simulink model "pct23_mpc_ref_tracking_anti_windup_notworking"  (R2020b)
settings: Solver=FixedStepAuto  StartTime=0.0  StopTime=6000  FixedStep=Ts  RelTol=1e-3
values from neighbouring files (symbols this model uses):
  cit = cit{1}    [mpc_init.m]    (also in mpc_init_reference_tracking_tunable.m; ref_tracking1.mat = [0 0.565401791493]; ref_tracking10.mat = [0 0.565401791493]; ref_tracking11.mat = [0 0.565401791493])
  men = men{1}    [mpc_init.m]    (also in mpc_init_reference_tracking_tunable.m; ref_tracking1.mat = [1 -0.434598208507]; ref_tracking10.mat = [1 -0.434598208507]; ref_tracking11.mat = [1 -0.434598208507])
  Ts = 0.5    [mpc_init.m]    (also in mpc_init_reference_tracking_tunable.m; mpc_modif.m = 1; mpc_original.m; ref_tracking1.mat)
  ts = 0.5    [mpc_init.m]    (also in mpc_init_reference_tracking_tunable.m = 1; mpc_modif.m = 1; mpc_original.m = 1; ref_tracking1.mat)
  us = 35    [mpc_init.m]    (also in mpc_init_reference_tracking_tunable.m; mpc_modif.m = 50; mpc_original.m = 50; ref_tracking1.mat)
  ys = 35    [mpc_init.m]    (also in mpc_init_reference_tracking_tunable.m; mpc_modif.m; mpc_original.m; ref_tracking1.mat)
undefined symbols (not defined in the file or in its folder): MPC_fcn_yref
libraries: pid_lib x1, pct23_lib x1
settings Model: EnablePacing=on  Creator=belko  LastModifiedBy=lgalc

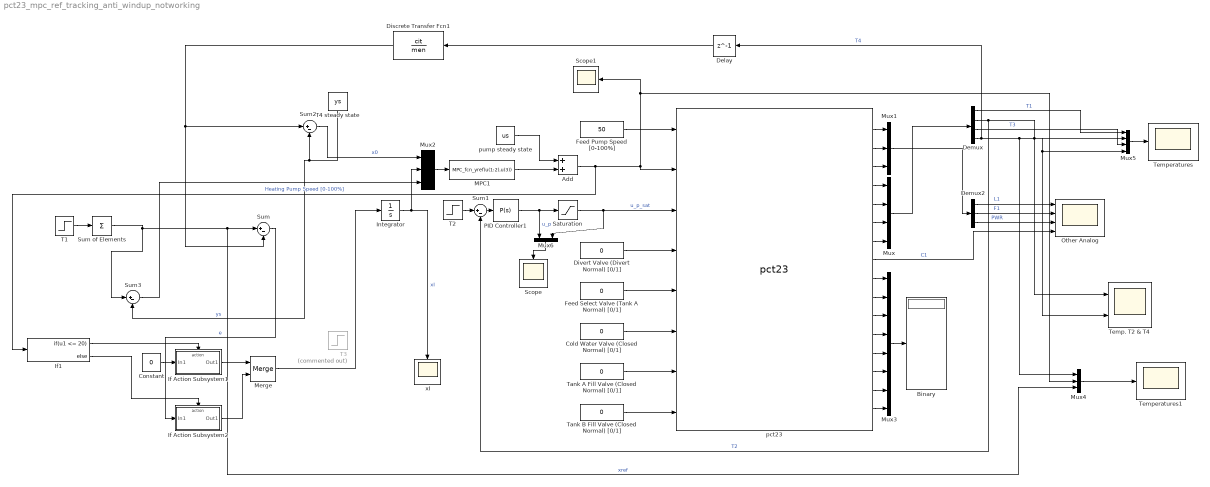
== system pct23_mpc_ref_tracking_anti_windup_notworking ==
  Add : Sum
  Binary : Display
  Cold Water Valve (Closed Normal) [0/1] : Constant  Value=0
  Constant : Constant  Value=0
  Delay : Delay  DelayLength=1  InitialCondition=ys  SampleTime=Ts
  Demux : Demux
  Demux2 : Demux  Outputs=3
  Discrete Transfer Fcn1 : DiscreteTransferFcn  Numerator=cit  Denominator=men  SampleTime=Ts
  Divert Valve (Divert Normal) [0/1] : Constant  Value=0
  Feed Pump Speed [0-100%] : Constant  Value=50
  Feed Select Valve (Tank A Normal) [0/1] : Constant  Value=0
  If Action Subsystem1 : Subsystem  TreatAsAtomicUnit=on
  If Action Subsystem2 : Subsystem  TreatAsAtomicUnit=on
  If1 : If  IfExpression=u1 <= 20
  Integrator : Integrator
  MPC1 : MATLABFcn  MATLABFcn=MPC_fcn_yref(u(1:2),u(3))  SampleTime=ts
  Merge : Merge  InitialOutput=0
  Mux : Mux
  Mux1 : Mux  Inputs=3
  Mux2 : Mux  Inputs=3
  Mux3 : Mux  Inputs=8
  Mux4 : Mux  Inputs=3
  Mux5 : Mux
  Mux6 : Mux  Inputs=2
  Other Analog : Scope  NumInputPorts=4
  PID Controller1 : pid_lib/PID Controller  Controller=P  Form=Parallel  TimeDomain=Continuous-time  UseExternalTs=off  SampleTime=-1  IntegratorMethod=Forward Euler  FilterMethod=Forward Euler  ControllerParametersSource=internal  P=20  I=1  D=0  UseFilter=on  N=100  TunerSelectOption=Transfer Function Based (PID Tuner App)  InitialConditionSource=internal  InitialConditionForIntegrator=0  InitialConditionForFilter=0  DifferentiatorICPrevScaledInput=0  ExternalReset=none  TrackingMode=off  Kt=1  LimitOutput=off  SatLimitsSource=internal  UpperSaturationLimit=inf  LowerSaturationLimit=-inf  LinearizeAsGain=on  AntiWindupMode=none  Kb=1  POutMin=[]  POutMax=[]  IOutMin=[]  IOutMax=[]  DOutMin=[]  DOutMax=[]  NOutMin=[]  NOutMax=[]  SumOutMin=[]  SumOutMax=[]  SaturationOutMin=[]  SaturationOutMax=[]  PParamMin=[]  PParamMax=[]  IParamMin=[]  IParamMax=[]  DParamMin=[]  DParamMax=[]  NParamMin=[]  NParamMax=[]  KbParamMin=[]  KbParamMax=[]  KtParamMin=[]  KtParamMax=[]  KbOutMin=[]  KbOutMax=[]  KtOutMin=[]  KtOutMax=[]  IntegratorOutMin=[]  IntegratorOutMax=[]  FilterOutMin=[]  FilterOutMax=[]  SumI1OutMin=[]  SumI1OutMax=[]  SumI2OutMin=[]  SumI2OutMax=[]  SumI3OutMin=[]  SumI3OutMax=[]  SumI4OutMin=[]  SumI4OutMax=[]  SumDOutMin=[]  SumDOutMax=[]  DifferentiatorOutMin=[]  DifferentiatorOutMax=[]  FilterDiffOutCoefMin=[]  FilterDiffOutCoefMax=[]  ReciprocalOutMin=[]  ReciprocalOutMax=[]  SumDenOutMin=[]  SumDenOutMax=[]  SumNumOutMin=[]  SumNumOutMax=[]  DivideOutMin=[]  DivideOutMax=[]  UdiffTsProdOutMin=[]  UdiffTsProdOutMax=[]  NTsProdOutMin=[]  NTsProdOutMax=[]  UintegralTsProdOutMin=[]  UintegralTsProdOutMax=[]  UngainTsProdOutMin=[]  UngainTsProdOutMax=[]  IntegratorContinuousStateAttributes=''  IntegratorStateMustResolveToSignalObject=off  IntegratorRTWStateStorageClass=Auto  FilterContinuousStateAttributes=''  FilterStateMustResolveToSignalObject=off  FilterRTWStateStorageClass=Auto  ParallelPVariant=InternalParameters  IdealPVariant=Disabled  IVariant=Disabled  DVariant=Disabled  IntegratorVariant=Disabled  SatVariant=Disabled  AWVariant=Disabled  PCopyVariant=Disabled  TRVariant=Disabled  FdbkBlocksVariant=Forward  IdealPFdbkVariant=Disabled  SatFdbkVariant=Disabled  DerivativeFilterVariant=Disabled  NVariant=Disabled  NCopyVariant=Disabled_SignalSpec  FilterICVariant=Disabled  IntegratorICVariant=Disabled  ExternalResetVariant=Disabled  TRSumVariant=Passthrough  SumFdbkVariant=Disabled  SumVariant=Passthrough_P  TsampFilterVariant=InternalTs  TsampNgainVariant=Passthrough  TsampIntegralVariant=Disabled_SignalSpec  ExternalSaturationOutDataTypeStr=Inherit: Same as second input
  Saturation : Saturate  UpperLimit=100  LowerLimit=0
  Scope : Scope
  Scope1 : Scope
  Sum{,1..3} (4 alike) : Sum  Inputs=|+-
  Sum of Elements : Sum  Inputs=+
  T1 : Step  Time=[1000 2000 3000 4000]  Before=[ys 0 0 0]  After=[ys+10, 5, -5, -10]  SampleTime=0
  T2 : Step  Time=0  Before=71  After=71  SampleTime=0
  T3 : Step  Commented=on  Time=[1000 2000 3000]  Before=[ys+15 0 0]  After=[ys+5, -5, -5]  SampleTime=0
  T4 steady state : Constant  Value=ys
  Tank A Fill Valve (Closed Normal) [0/1] : Constant  Value=0
  Tank B Fill Valve (Closed Normal) [0/1] : Constant  Value=0
  Temp. T2 & T4 : Scope  NumInputPorts=2
  Temperatures : Scope
  Temperatures1 : Scope
  pct23 : pct23_lib/pct23  SystemSampleTime=-1  VariantActivationTime=update diagram  Latency=0  AutoFrameSizeCalculation=off
  pump steady state : Constant  Value=us
  xI : Scope
  wires:
  Sum1/1 -> PID Controller1/1
  pct23/12 -> Mux3/4
  Tank B Fill Valve (Closed Normal) [0/1]/1 -> pct23/8
  MPC1/1 -> Add/2
  pct23/1 -> Mux1/1
  Mux6/1 -> Scope/1
  Mux5/1 -> Temperatures/1
  Tank A Fill Valve (Closed Normal) [0/1]/1 -> pct23/7
  PID Controller1/1 -> Mux6/1, Saturation/1  "u_p"
  pct23/15 -> Mux3/7
  T2/1 -> Sum1/1
  Demux/3 -> Mux5/3  "T3"
  Add/1 -> If1/1, pct23/2, Mux4/2, Scope1/1  "Heating Pump Speed [0-100%]"
  Demux2/1 -> Other Analog/1  "L1"
  pct23/10 -> Mux3/2
  pct23/8 -> Other Analog/4  "C1"
  pump steady state/1 -> Add/1
  Delay/1 -> Discrete Transfer Fcn1/1
  Saturation/1 -> pct23/3, Mux6/2  "u_p_sat"
  pct23/2 -> Mux1/2
  pct23/11 -> Mux3/3
  Feed Pump Speed [0-100%]/1 -> pct23/1
  T1/1 -> Sum of Elements/1
  Feed Select Valve (Tank A Normal) [0/1]/1 -> pct23/5
  pct23/4 -> Mux/1
  pct23/13 -> Mux3/5
  Demux2/3 -> Other Analog/3  "PWR"
  Mux3/1 -> Binary/1
  Mux4/1 -> Temperatures1/1
  pct23/3 -> Mux1/3
  Sum of Elements/1 -> Mux4/3, Sum/1, Sum3/1  "xref"
  pct23/9 -> Mux3/1
  Divert Valve (Divert Normal) [0/1]/1 -> pct23/4
  T4 steady state/1 -> Sum3/2, Sum2/2  "ys"
  Mux1/1 -> Demux2/1
  Demux/1 -> Mux5/1  "T1"
  pct23/14 -> Mux3/6
  Sum2/1 -> Mux2/1  "x0"
  pct23/16 -> Mux3/8
  Cold Water Valve (Closed Normal) [0/1]/1 -> pct23/6
  pct23/6 -> Mux/3
  Mux/1 -> Demux/1
  Demux2/2 -> Other Analog/2  "F1"
  Demux/4 -> Mux4/1, Temp. T2 & T4/2, Mux5/4, Delay/1  "T4"
  pct23/5 -> Mux/2
  pct23/7 -> Mux/4
  Demux/2 -> Temp. T2 & T4/1, Mux5/2, Sum1/2  "T2"
  Mux2/1 -> MPC1/1
  Sum3/1 -> Mux2/3
  Integrator/1 -> Mux2/2, xI/1  "xI"
  If Action Subsystem1/1(Out1) -> Merge/1
  Constant/1 -> If Action Subsystem1/1(In1)
  Sum/1 -> If Action Subsystem2/1(In1)  "e"
  If1/1 -> If Action Subsystem1/Action
  If1/2 -> If Action Subsystem2/Action
  If Action Subsystem2/1(Out1) -> Merge/2
  Discrete Transfer Fcn1/1 -> Sum2/1, Sum/2
  Merge/1 -> Integrator/1

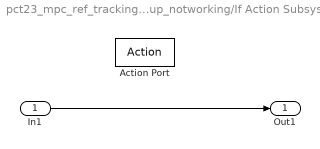
== system pct23_mpc_ref_tracking_anti_windup_notworking/If Action Subsystem1 ==
  In1 : Inport
  Action Port : ActionPort  ActionPortLabel=if(u1 <= 20)
  Out1 : Outport
  wires:
  In1/1 -> Out1/1

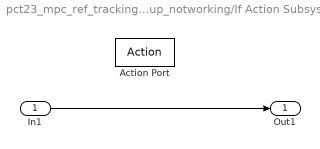
== system pct23_mpc_ref_tracking_anti_windup_notworking/If Action Subsystem2 ==
  In1 : Inport
  Action Port : ActionPort  ActionPortLabel=else
  Out1 : Outport
  wires:
  In1/1 -> Out1/1
